simulink model "coefficent_aray"  (R2024a)
settings: Solver=FixedStepDiscrete  StartTime=0.0  StopTime=0.001  RelTol=1e-3
values from neighbouring files (symbols this model uses):
  Ts = 1/Fs    (= 7.50007500075e-06)    [new_generation_coeff.m]    (also in simon_test.m; simple_fft_test.m = 1/F; testPSD_c2d.m; testPSD_simulink.m)
settings Model: DataTypeOverride=Off  Creator=Simon  LastModifiedBy=Simon
settings OptimizationCC: BlockReduction=off  ConditionallyExecuteInputs=off  DefaultParameterBehavior=Inlined  InheritOutputTypeSmallerThanSingle=on
settings DebuggingCC: AlgebraicLoopMsg=error  SingleTaskRateTransMsg=error  UnconnectedInputMsg=warning  UnconnectedOutputMsg=warning  UnconnectedLineMsg=warning
settings HardwareCC: ProdBitPerPointer=32  ProdBitPerSizeT=32  ProdBitPerPtrDiffT=32  ProdLargestAtomicFloat=None  ProdIntDivRoundTo=Undefined  ProdEndianess=Unspecified  ProdWordSize=32  ProdHWDeviceType=ASIC/FPGA->ASIC/FPGA  TargetBitPerPointer=64  TargetBitPerSizeT=64  TargetBitPerPtrDiffT=64  TargetLongLongMode=on  TargetIntDivRoundTo=Zero  TargetEndianess=LittleEndian  TargetWordSize=64  TargetHWDeviceType=Custom Processor->MATLAB Host Computer  ProdEqTarget=off

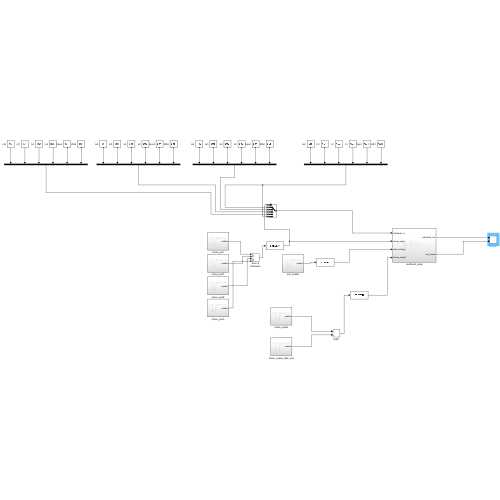
[thumbnail: Simulink's stored preview of the top-level diagram]
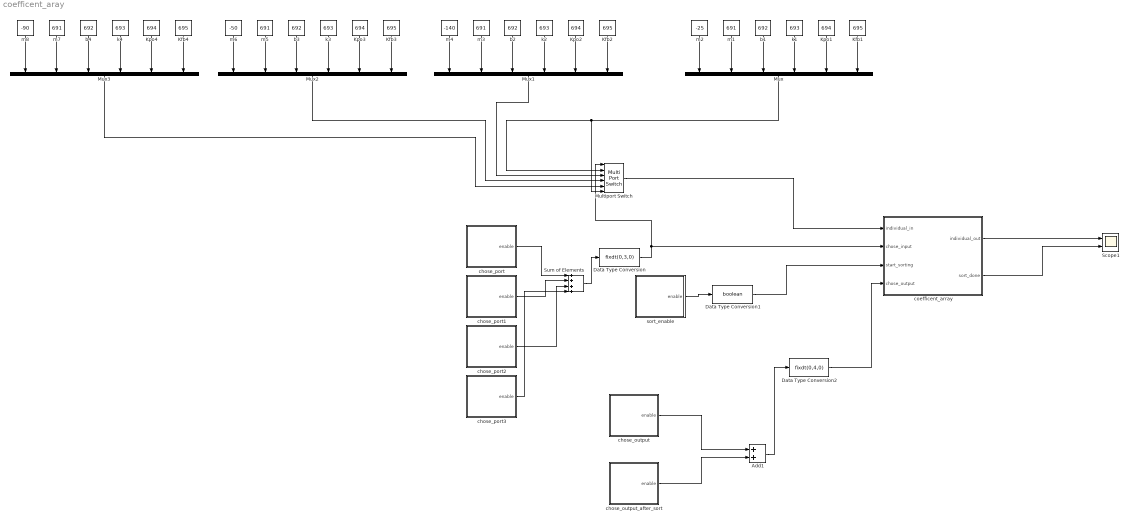
== system coefficent_aray ==
  Add1 : Sum
  Data Type Conversion : DataTypeConversion  OutDataTypeStr=fixdt(0,3,0)  SaturateOnIntegerOverflow=off  RndMeth=Floor
  Data Type Conversion1 : DataTypeConversion  OutDataTypeStr=boolean  SaturateOnIntegerOverflow=off  RndMeth=Floor
  Data Type Conversion2 : DataTypeConversion  OutDataTypeStr=fixdt(0,4,0)  SaturateOnIntegerOverflow=off  RndMeth=Floor
  Kfb{1..4} (4 alike) : Constant  Value=695  OutDataTypeStr=fixdt(1,64,32)  SampleTime=Ts
  Kpo{1..4} (4 alike) : Constant  Value=694  OutDataTypeStr=fixdt(1,64,32)  SampleTime=Ts
  Multiport Switch : MultiPortSwitch  Inputs=4  DataPortForDefault=Additional data port  DiagnosticForDefault=None  SaturateOnIntegerOverflow=off  InputSameDT=off
  Mux{,1..3} (4 alike) : Mux  Inputs=6
  Scope1 : Scope  NumInputPorts=2
  Sum of Elements : Sum  Inputs=++++
  b{1..4} (4 alike) : Constant  Value=692  OutDataTypeStr=fixdt(1,64,32)  SampleTime=Ts
  chose_output : Subsystem
  chose_output_after_sort : Subsystem
  chose_port : Subsystem
  chose_port1 : Subsystem
  chose_port2 : Subsystem
  chose_port3 : Subsystem
  coefficent_array : Subsystem
  k{1..4} (4 alike) : Constant  Value=693  OutDataTypeStr=fixdt(1,64,32)  SampleTime=Ts
  m{1,3,5,7} (4 alike) : Constant  Value=691  OutDataTypeStr=fixdt(1,64,32)  SampleTime=Ts
  m2 : Constant  Value=-25  OutDataTypeStr=fixdt(1,64,32)  SampleTime=Ts
  m4 : Constant  Value=-140  OutDataTypeStr=fixdt(1,64,32)  SampleTime=Ts
  m6 : Constant  Value=-50  OutDataTypeStr=fixdt(1,64,32)  SampleTime=Ts
  m8 : Constant  Value=-90  OutDataTypeStr=fixdt(1,64,32)  SampleTime=Ts
  sort_enable : Subsystem
  wires:
  Kpo1/1 -> Mux/5
  Kfb1/1 -> Mux/6
  k1/1 -> Mux/4
  m1/1 -> Mux/2
  b1/1 -> Mux/3
  m2/1 -> Mux/1
  chose_output/1(enable) -> Add1/1
  chose_output_after_sort/1(enable) -> Add1/2
  coefficent_array/1(individual_out) -> Scope1/1
  coefficent_array/2(sort_done) -> Scope1/2
  Kpo2/1 -> Mux1/5
  b2/1 -> Mux1/3
  k2/1 -> Mux1/4
  Kfb2/1 -> Mux1/6
  m4/1 -> Mux1/1
  m3/1 -> Mux1/2
  Kpo3/1 -> Mux2/5
  b3/1 -> Mux2/3
  k3/1 -> Mux2/4
  Kfb3/1 -> Mux2/6
  m6/1 -> Mux2/1
  m5/1 -> Mux2/2
  Kpo4/1 -> Mux3/5
  b4/1 -> Mux3/3
  k4/1 -> Mux3/4
  Kfb4/1 -> Mux3/6
  m8/1 -> Mux3/1
  m7/1 -> Mux3/2
  Multiport Switch/1 -> coefficent_array/1(individual_in)
  Mux/1 -> Multiport Switch/6, Multiport Switch/2
  Mux1/1 -> Multiport Switch/3
  Mux2/1 -> Multiport Switch/4
  Mux3/1 -> Multiport Switch/5
  chose_port/1(enable) -> Sum of Elements/1
  chose_port1/1(enable) -> Sum of Elements/2
  chose_port2/1(enable) -> Sum of Elements/3
  chose_port3/1(enable) -> Sum of Elements/4
  Add1/1 -> Data Type Conversion2/1
  sort_enable/1(enable) -> Data Type Conversion1/1
  Data Type Conversion/1 -> coefficent_array/2(chose_input), Multiport Switch/1
  Data Type Conversion1/1 -> coefficent_array/3(start_sorting)
  Data Type Conversion2/1 -> coefficent_array/4(chose_output)
  Sum of Elements/1 -> Data Type Conversion/1

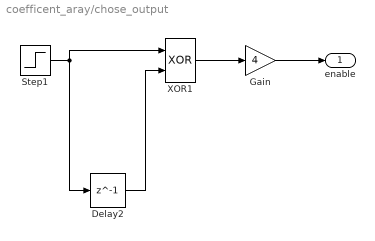
== system coefficent_aray/chose_output ==
  Delay2 : Delay  DelayLength=1  InitialCondition=0  SampleTime=Ts
  Gain : Gain  Gain=4
  Step1 : Step  Time=Ts*15  SampleTime=Ts
  XOR1 : Logic  Operator=XOR  IconShape=distinctive  AllPortsSameDT=off  OutDataTypeStr=fixdt(0,8)
  enable : Outport
  wires:
  XOR1/1 -> Gain/1
  Step1/1 -> Delay2/1, XOR1/1
  Delay2/1 -> XOR1/2
  Gain/1 -> enable/1

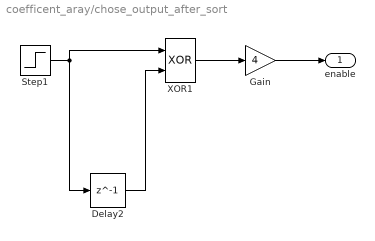
== system coefficent_aray/chose_output_after_sort ==
  Delay2 : Delay  DelayLength=1  InitialCondition=0  SampleTime=Ts
  Gain : Gain  Gain=4
  Step1 : Step  Time=Ts*50  SampleTime=Ts
  XOR1 : Logic  Operator=XOR  IconShape=distinctive  AllPortsSameDT=off  OutDataTypeStr=fixdt(0,8)
  enable : Outport
  wires:
  XOR1/1 -> Gain/1
  Step1/1 -> Delay2/1, XOR1/1
  Delay2/1 -> XOR1/2
  Gain/1 -> enable/1

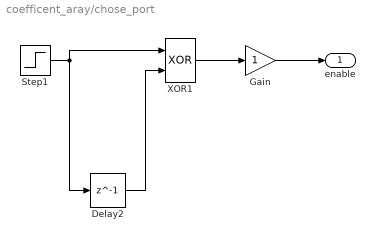
== system coefficent_aray/chose_port ==
  Delay2 : Delay  DelayLength=1  InitialCondition=0  SampleTime=Ts
  Gain : Gain
  Step1 : Step  Time=Ts*5  SampleTime=Ts
  XOR1 : Logic  Operator=XOR  IconShape=distinctive  AllPortsSameDT=off  OutDataTypeStr=fixdt(0,8)
  enable : Outport
  wires:
  XOR1/1 -> Gain/1
  Step1/1 -> Delay2/1, XOR1/1
  Delay2/1 -> XOR1/2
  Gain/1 -> enable/1

== system coefficent_aray/chose_port1 ==
  Delay2 : Delay  DelayLength=1  InitialCondition=0  SampleTime=Ts
  Gain : Gain  Gain=2
  Step1 : Step  Time=Ts*7  SampleTime=Ts
  XOR1 : Logic  Operator=XOR  IconShape=distinctive  AllPortsSameDT=off  OutDataTypeStr=fixdt(0,8)
  enable : Outport
  wires:
  XOR1/1 -> Gain/1
  Step1/1 -> Delay2/1, XOR1/1
  Delay2/1 -> XOR1/2
  Gain/1 -> enable/1

== system coefficent_aray/chose_port2 ==
  Delay2 : Delay  DelayLength=1  InitialCondition=0  SampleTime=Ts
  Gain : Gain  Gain=3
  Step1 : Step  Time=Ts*9  SampleTime=Ts
  XOR1 : Logic  Operator=XOR  IconShape=distinctive  AllPortsSameDT=off  OutDataTypeStr=fixdt(0,8)
  enable : Outport
  wires:
  XOR1/1 -> Gain/1
  Step1/1 -> Delay2/1, XOR1/1
  Delay2/1 -> XOR1/2
  Gain/1 -> enable/1

== system coefficent_aray/chose_port3 ==
  Delay2 : Delay  DelayLength=1  InitialCondition=0  SampleTime=Ts
  Gain : Gain  Gain=4
  Step1 : Step  Time=Ts*11  SampleTime=Ts
  XOR1 : Logic  Operator=XOR  IconShape=distinctive  AllPortsSameDT=off  OutDataTypeStr=fixdt(0,8)
  enable : Outport
  wires:
  XOR1/1 -> Gain/1
  Step1/1 -> Delay2/1, XOR1/1
  Delay2/1 -> XOR1/2
  Gain/1 -> enable/1

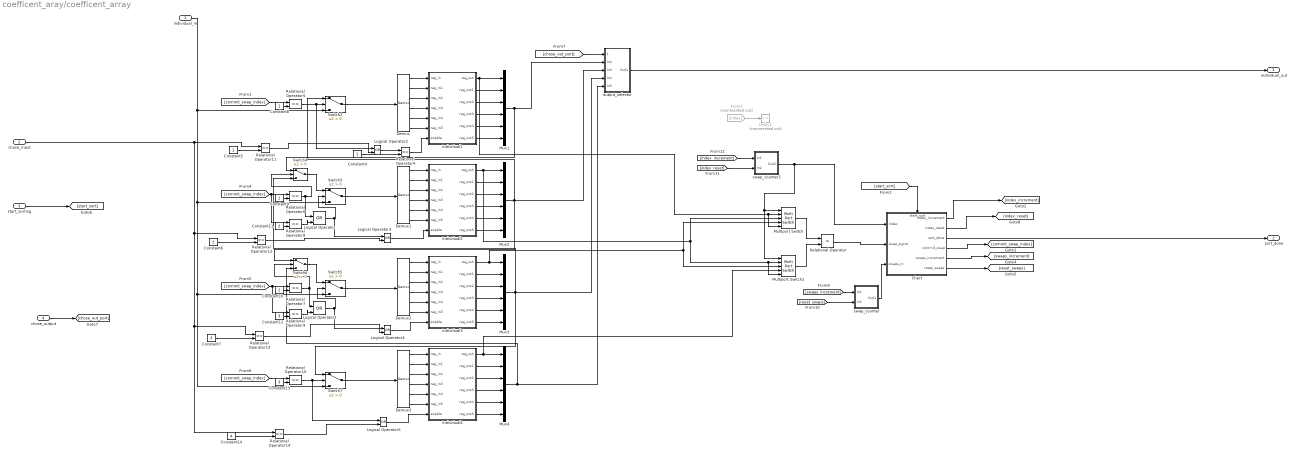
== system coefficent_aray/coefficent_array ==
  individual_in : Inport
  chose_input : Inport  Port=2
  start_sorting : Inport  Port=3
  chose_output : Inport  Port=4
  Chart : Stateflow chart  TreatAsAtomicUnit=on
      settings: PortSchema="{\"entries\":[{\"content\":{\"sides\":[{\"content\":{\"connectorIds\":[\"In1\",\"In4\",\"In3\"]},\"type\":\"ConnectorPlacement.EquallySpacedRectSide\",\"uuid\":\"bd2dafac-a5a9-4836-b8bd-cefb36fb6626\"},{\"content\":{\"connectorIds\":[\"Out1\",\"Out2\",\"Out3\",\"Out4\",\"Out5\",\"Out6\"],\"side\":\"RIGHT\"},\"type\":\"ConnectorPlacement.EquallySpacedRectSide\",\"uuid\":\"b2eb894e-8d56-4038-acbe-51c43d919a15\"},{\"content\":{\"connectorIds\":[\"In2\"],\"side\":\"TOP\"},\"type\":\"ConnectorPlacement.EquallySpacedRectSide\",\"uuid\":\"645ecb99-1eca-4a2d-8e44-d34ac75e3d1a\"}]},\"type\":\"ConnectorPlacement.EquallySpacedConnector\",\"uuid\":\"63f53eab-c5ec-482c-b992-d953653b0c27\"}],\"packageUris\":[\"http://schema.mathworks.com/mf0/Connector/R2020b\"],\"version\":\"1.0\"}"
  Constant10 : Constant  Value=2  OutDataTypeStr=fixdt(0,4,0)  SampleTime=Ts
  Constant11 : Constant  Value=2  OutDataTypeStr=fixdt(0,4,0)  SampleTime=Ts
  Constant12 : Constant  Value=3  OutDataTypeStr=fixdt(0,4,0)  SampleTime=Ts
  Constant13 : Constant  Value=3  OutDataTypeStr=fixdt(0,4,0)  SampleTime=Ts
  Constant14 : Constant  Value=4  OutDataTypeStr=fixdt(0,4,0)  SampleTime=Ts
  Constant{4..5,8..9} (4 alike) : Constant  OutDataTypeStr=fixdt(0,4,0)  SampleTime=Ts
  Constant6 : Constant  Value=2  OutDataTypeStr=fixdt(0,4,0)  SampleTime=Ts
  Constant7 : Constant  Value=3  OutDataTypeStr=fixdt(0,4,0)  SampleTime=Ts
  Delay1 : Delay  Commented=on  DelayLength=1  InitialCondition=0
  Demux{,1..3} (4 alike) : Demux  Outputs=6
  From3 : From  Commented=on  GotoTag=index
  Logical Operator{,1..5} (6 alike) : Logic  Operator=OR  IconShape=distinctive  AllPortsSameDT=off  OutDataTypeStr=boolean
  Multiport Switch : MultiPortSwitch  DataPortForDefault=Additional data port  DiagnosticForDefault=None  SaturateOnIntegerOverflow=off  InputSameDT=off
  Multiport Switch1 : MultiPortSwitch  DataPortForDefault=Additional data port  DiagnosticForDefault=None  SaturateOnIntegerOverflow=off  InputSameDT=off
  Mux{1..4} (4 alike) : Mux  Inputs=6
  Relational Operator : RelationalOperator  Operator=>  OutDataTypeStr=boolean  InputSameDT=off
  Relational Operator{4..14} (11 alike) : RelationalOperator  Operator===  OutDataTypeStr=boolean  RndMeth=Simplest  InputSameDT=off
  Switch{2..7} (6 alike) : Switch  Criteria=u2 > Threshold  SaturateOnIntegerOverflow=off  InputSameDT=off
  individual1 : Subsystem
  individual2 : Subsystem
  individual3 : Subsystem
  individual4 : Subsystem
  output_selector : Subsystem
  swap_counter : Subsystem
  swap_counter1 : Subsystem
  individual_out : Outport
  sort_done : Outport  Port=2
  wires:
  Logical Operator1/1 -> Logical Operator4/1, Switch5/2
  individual3/6(reg_out5) -> Mux3/6
  Constant9/1 -> Relational Operator6/2
  individual2/6(reg_out5) -> Mux2/6
  Demux2/3 -> individual3/3(reg_in2)
  Chart/5(swaps_increment) -> [swaps_increment]
  swap_counter1/1(Out1) -> Multiport Switch1/1, Multiport Switch/1, Chart/1(index)
  Switch4/1 -> Switch3/1
  individual1/1(reg_out) -> Mux1/1, Multiport Switch/5, Multiport Switch/2
  Demux/1 -> individual1/1(reg_in)
  Mux3/1 -> output_selector/4(In4), Switch7/1, Switch4/3
  individual3/3(reg_out2) -> Mux3/3
  individual4/4(reg_out3) -> Mux4/4
  Relational Operator10/1 -> Logical Operator5/1, Switch7/2
  [reset_swaps] -> swap_counter/2(In2)
  swap_counter/1(Out1) -> Chart/3(swaps_in)
  individual1/3(reg_out2) -> Mux1/3
  Relational Operator5/1 -> Logical Operator2/1, Switch2/2
  [swaps_increment] -> swap_counter/1(In1)
  [commit_swap_index] -> Relational Operator5/1
  Demux3/1 -> individual4/1(reg_in)
  Demux3/6 -> individual4/6(reg_in5)
  individual4/6(reg_out5) -> Mux4/6
  Demux1/4 -> individual2/4(reg_in3)
  Mux1/1 -> Switch4/1, output_selector/2(In2)
  Chart/6(reset_swaps) -> [reset_swaps]
  Relational Operator8/1 -> Logical Operator/2
  [commit_swap_index] -> Relational Operator8/1, Relational Operator6/1
  individual4/3(reg_out2) -> Mux4/3
  [commit_swap_index] -> Relational Operator9/1, Relational Operator7/1
  Logical Operator3/1 -> individual2/7(enable)
  Logical Operator5/1 -> individual4/7(enable)
  Multiport Switch/1 -> Relational Operator/1
  Constant11/1 -> Relational Operator8/2
  start_sorting/1 -> [start_sort]
  Chart/4(commit_swap) -> [commit_swap_index]
  Logical Operator/1 -> Logical Operator3/1, Switch3/2
  Demux/5 -> individual1/5(reg_in4)
  individual_in/1 -> Switch7/3, Switch5/3, Switch3/3, Switch2/3
  Demux2/1 -> individual3/1(reg_in)
  Switch3/1 -> Demux1/1
  individual4/1(reg_out) -> Multiport Switch1/4, Mux4/1
  Relational Operator6/1 -> Logical Operator/1, Switch4/2
  Constant4/1 -> Relational Operator4/2
  Constant13/1 -> Relational Operator10/2
  Constant12/1 -> Relational Operator9/2
  [commit_swap_index] -> Relational Operator10/1
  Demux2/4 -> individual3/4(reg_in3)
  individual2/4(reg_out3) -> Mux2/4
  Demux2/6 -> individual3/6(reg_in5)
  Demux1/6 -> individual2/6(reg_in5)
  Switch6/1 -> Switch5/1
  output_selector/1(Out1) -> individual_out/1
  Demux2/2 -> individual3/2(reg_in1)
  individual2/1(reg_out) -> Multiport Switch/3, Multiport Switch1/5, Multiport Switch1/2, Mux2/1
  Demux1/2 -> individual2/2(reg_in1)
  [chose_out_port] -> output_selector/1(chose_port)
  individual3/5(reg_out4) -> Mux3/5
  Demux/6 -> individual1/6(reg_in5)
  individual4/2(reg_out1) -> Mux4/2
  individual3/4(reg_out3) -> Mux3/4
  chose_input/1 -> Relational Operator14/1, Relational Operator13/1, Relational Operator12/1, Relational Operator11/1
  Relational Operator/1 -> Chart/4(swap_signal)
  Demux2/5 -> individual3/5(reg_in4)
  Logical Operator4/1 -> individual3/7(enable)
  Demux/3 -> individual1/3(reg_in2)
  Demux3/5 -> individual4/5(reg_in4)
  Demux3/4 -> individual4/4(reg_in3)
  Mux4/1 -> Switch6/3, output_selector/5(In5)
  Mux2/1 -> output_selector/3(In3), Switch6/1, Switch2/1
  individual3/1(reg_out) -> Multiport Switch1/3, Multiport Switch/4, Mux3/1
  individual4/5(reg_out4) -> Mux4/5
  individual3/2(reg_out1) -> Mux3/2
  individual2/5(reg_out4) -> Mux2/5
  Constant8/1 -> Relational Operator5/2
  Switch7/1 -> Demux3/1
  Chart/1(index_increment) -> [index_increment]
  Switch5/1 -> Demux2/1
  Demux3/2 -> individual4/2(reg_in1)
  individual2/2(reg_out1) -> Mux2/2
  Relational Operator7/1 -> Logical Operator1/1, Switch6/2
  Multiport Switch1/1 -> Relational Operator/2
  Demux1/5 -> individual2/5(reg_in4)
  Switch2/1 -> Demux/1
  Demux3/3 -> individual4/3(reg_in2)
  Relational Operator9/1 -> Logical Operator1/2
  Constant10/1 -> Relational Operator7/2
  Logical Operator2/1 -> Relational Operator4/1
  individual1/5(reg_out4) -> Mux1/5
  Demux/2 -> individual1/2(reg_in1)
  individual1/6(reg_out5) -> Mux1/6
  Relational Operator4/1 -> individual1/7(enable)
  individual1/2(reg_out1) -> Mux1/2
  Demux/4 -> individual1/4(reg_in3)
  Demux1/3 -> individual2/3(reg_in2)
  individual1/4(reg_out3) -> Mux1/4
  individual2/3(reg_out2) -> Mux2/3
  Demux1/1 -> individual2/1(reg_in)
  [start_sort] -> Chart/2(start_sort)
  Chart/3(sort_done) -> sort_done/1
  chose_output/1 -> [chose_out_port]
  Constant5/1 -> Relational Operator11/2
  Relational Operator11/1 -> Logical Operator2/2
  Constant6/1 -> Relational Operator12/2
  Relational Operator12/1 -> Logical Operator3/2
  Constant7/1 -> Relational Operator13/2
  Relational Operator13/1 -> Logical Operator4/2
  Relational Operator14/1 -> Logical Operator5/2
  Constant14/1 -> Relational Operator14/2
  [index_increment] -> swap_counter1/1(In1)
  [index_reset] -> swap_counter1/2(In2)
  From3/1 -> Delay1/1
  Chart/2(index_reset) -> [index_reset]

== system coefficent_aray/sort_enable ==
  Delay2 : Delay  DelayLength=1  InitialCondition=0  SampleTime=Ts
  Gain : Gain
  Step1 : Step  Time=Ts*20  SampleTime=Ts
  XOR1 : Logic  Operator=XOR  IconShape=distinctive  AllPortsSameDT=off  OutDataTypeStr=fixdt(0,8)
  enable : Outport
  wires:
  XOR1/1 -> Gain/1
  Step1/1 -> Delay2/1, XOR1/1
  Delay2/1 -> XOR1/2
  Gain/1 -> enable/1

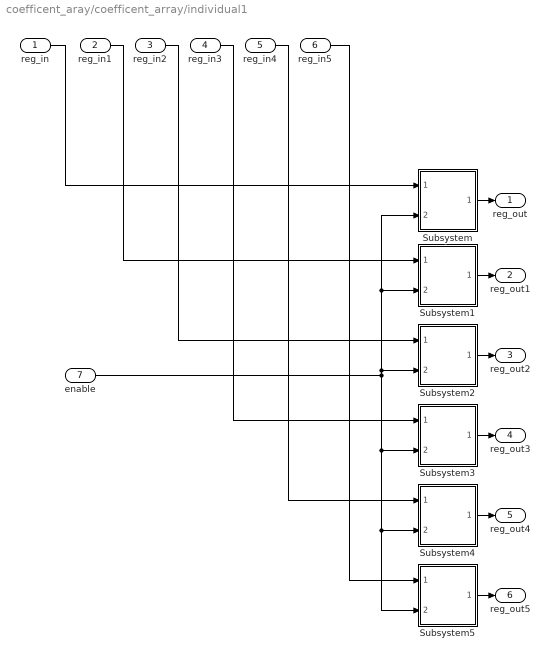
== system coefficent_aray/coefficent_array/individual1 ==
  reg_in : Inport
  reg_in1 : Inport  Port=2
  reg_in2 : Inport  Port=3
  reg_in3 : Inport  Port=4
  reg_in4 : Inport  Port=5
  reg_in5 : Inport  Port=6
  enable : Inport  Port=7
  Subsystem : Subsystem
  Subsystem1 : Subsystem
  Subsystem2 : Subsystem
  Subsystem3 : Subsystem
  Subsystem4 : Subsystem
  Subsystem5 : Subsystem
  reg_out : Outport
  reg_out1 : Outport  Port=2
  reg_out2 : Outport  Port=3
  reg_out3 : Outport  Port=4
  reg_out4 : Outport  Port=5
  reg_out5 : Outport  Port=6
  wires:
  enable/1 -> Subsystem2/2(enable), Subsystem1/2(enable), Subsystem/2(enable), Subsystem3/2(enable), Subsystem4/2(enable), Subsystem5/2(enable)
  Subsystem2/1(reg_out) -> reg_out2/1
  Subsystem4/1(reg_out) -> reg_out4/1
  Subsystem3/1(reg_out) -> reg_out3/1
  Subsystem1/1(reg_out) -> reg_out1/1
  reg_in/1 -> Subsystem/1(reg_in)
  Subsystem/1(reg_out) -> reg_out/1
  reg_in1/1 -> Subsystem1/1(reg_in)
  reg_in2/1 -> Subsystem2/1(reg_in)
  reg_in3/1 -> Subsystem3/1(reg_in)
  Subsystem5/1(reg_out) -> reg_out5/1
  reg_in4/1 -> Subsystem4/1(reg_in)
  reg_in5/1 -> Subsystem5/1(reg_in)

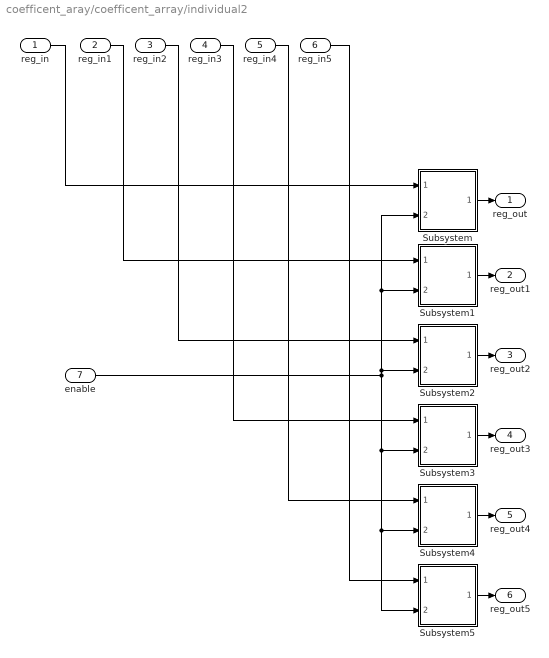
== system coefficent_aray/coefficent_array/individual2 ==
  reg_in : Inport
  reg_in1 : Inport  Port=2
  reg_in2 : Inport  Port=3
  reg_in3 : Inport  Port=4
  reg_in4 : Inport  Port=5
  reg_in5 : Inport  Port=6
  enable : Inport  Port=7
  Subsystem : Subsystem
  Subsystem1 : Subsystem
  Subsystem2 : Subsystem
  Subsystem3 : Subsystem
  Subsystem4 : Subsystem
  Subsystem5 : Subsystem
  reg_out : Outport
  reg_out1 : Outport  Port=2
  reg_out2 : Outport  Port=3
  reg_out3 : Outport  Port=4
  reg_out4 : Outport  Port=5
  reg_out5 : Outport  Port=6
  wires:
  enable/1 -> Subsystem2/2(enable), Subsystem1/2(enable), Subsystem/2(enable), Subsystem3/2(enable), Subsystem4/2(enable), Subsystem5/2(enable)
  Subsystem2/1(reg_out) -> reg_out2/1
  Subsystem4/1(reg_out) -> reg_out4/1
  Subsystem3/1(reg_out) -> reg_out3/1
  Subsystem1/1(reg_out) -> reg_out1/1
  reg_in/1 -> Subsystem/1(reg_in)
  Subsystem/1(reg_out) -> reg_out/1
  reg_in1/1 -> Subsystem1/1(reg_in)
  reg_in2/1 -> Subsystem2/1(reg_in)
  reg_in3/1 -> Subsystem3/1(reg_in)
  Subsystem5/1(reg_out) -> reg_out5/1
  reg_in4/1 -> Subsystem4/1(reg_in)
  reg_in5/1 -> Subsystem5/1(reg_in)

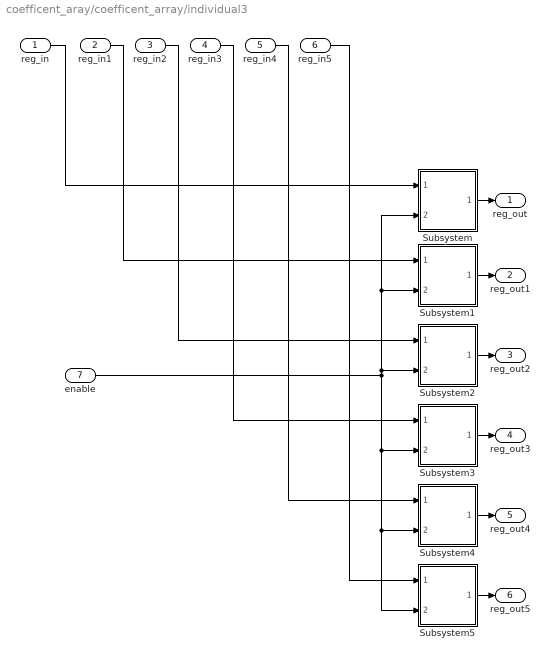
== system coefficent_aray/coefficent_array/individual3 ==
  reg_in : Inport
  reg_in1 : Inport  Port=2
  reg_in2 : Inport  Port=3
  reg_in3 : Inport  Port=4
  reg_in4 : Inport  Port=5
  reg_in5 : Inport  Port=6
  enable : Inport  Port=7
  Subsystem : Subsystem
  Subsystem1 : Subsystem
  Subsystem2 : Subsystem
  Subsystem3 : Subsystem
  Subsystem4 : Subsystem
  Subsystem5 : Subsystem
  reg_out : Outport
  reg_out1 : Outport  Port=2
  reg_out2 : Outport  Port=3
  reg_out3 : Outport  Port=4
  reg_out4 : Outport  Port=5
  reg_out5 : Outport  Port=6
  wires:
  enable/1 -> Subsystem2/2(enable), Subsystem1/2(enable), Subsystem/2(enable), Subsystem3/2(enable), Subsystem4/2(enable), Subsystem5/2(enable)
  Subsystem2/1(reg_out) -> reg_out2/1
  Subsystem4/1(reg_out) -> reg_out4/1
  Subsystem3/1(reg_out) -> reg_out3/1
  Subsystem1/1(reg_out) -> reg_out1/1
  reg_in/1 -> Subsystem/1(reg_in)
  Subsystem/1(reg_out) -> reg_out/1
  reg_in1/1 -> Subsystem1/1(reg_in)
  reg_in2/1 -> Subsystem2/1(reg_in)
  reg_in3/1 -> Subsystem3/1(reg_in)
  Subsystem5/1(reg_out) -> reg_out5/1
  reg_in4/1 -> Subsystem4/1(reg_in)
  reg_in5/1 -> Subsystem5/1(reg_in)

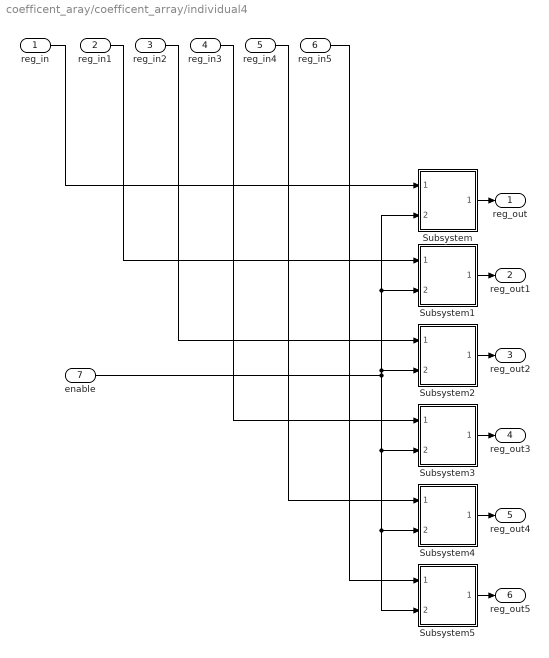
== system coefficent_aray/coefficent_array/individual4 ==
  reg_in : Inport
  reg_in1 : Inport  Port=2
  reg_in2 : Inport  Port=3
  reg_in3 : Inport  Port=4
  reg_in4 : Inport  Port=5
  reg_in5 : Inport  Port=6
  enable : Inport  Port=7
  Subsystem : Subsystem
  Subsystem1 : Subsystem
  Subsystem2 : Subsystem
  Subsystem3 : Subsystem
  Subsystem4 : Subsystem
  Subsystem5 : Subsystem
  reg_out : Outport
  reg_out1 : Outport  Port=2
  reg_out2 : Outport  Port=3
  reg_out3 : Outport  Port=4
  reg_out4 : Outport  Port=5
  reg_out5 : Outport  Port=6
  wires:
  enable/1 -> Subsystem2/2(enable), Subsystem1/2(enable), Subsystem/2(enable), Subsystem3/2(enable), Subsystem4/2(enable), Subsystem5/2(enable)
  Subsystem2/1(reg_out) -> reg_out2/1
  Subsystem4/1(reg_out) -> reg_out4/1
  Subsystem3/1(reg_out) -> reg_out3/1
  Subsystem1/1(reg_out) -> reg_out1/1
  reg_in/1 -> Subsystem/1(reg_in)
  Subsystem/1(reg_out) -> reg_out/1
  reg_in1/1 -> Subsystem1/1(reg_in)
  reg_in2/1 -> Subsystem2/1(reg_in)
  reg_in3/1 -> Subsystem3/1(reg_in)
  Subsystem5/1(reg_out) -> reg_out5/1
  reg_in4/1 -> Subsystem4/1(reg_in)
  reg_in5/1 -> Subsystem5/1(reg_in)

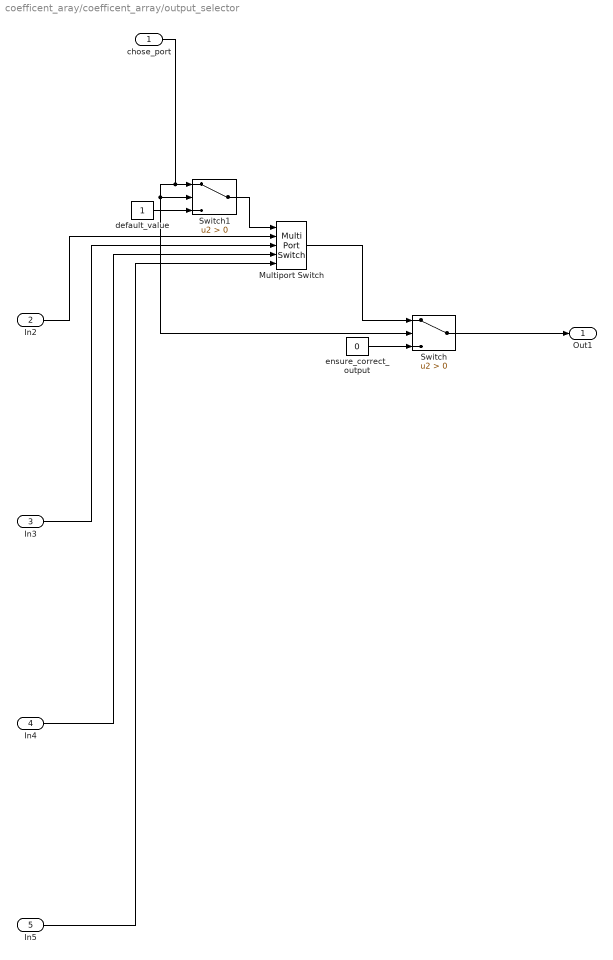
== system coefficent_aray/coefficent_array/output_selector ==
  chose_port : Inport
  In2 : Inport  Port=2
  In3 : Inport  Port=3
  In4 : Inport  Port=4
  In5 : Inport  Port=5
  Multiport Switch : MultiPortSwitch  Inputs=4  SaturateOnIntegerOverflow=off  InputSameDT=off
  Switch : Switch  Criteria=u2 > Threshold  SaturateOnIntegerOverflow=off  InputSameDT=off
  Switch1 : Switch  Criteria=u2 > Threshold  SaturateOnIntegerOverflow=off  InputSameDT=off
  default_value : Constant  OutDataTypeStr=fixdt(0,4,0)  SampleTime=Ts
  ensure_correct_output : Constant  Value=0  OutDataTypeStr=fixdt(0,1,0)  SampleTime=Ts
  Out1 : Outport
  wires:
  chose_port/1 -> Switch1/1, Switch/2, Switch1/2
  In2/1 -> Multiport Switch/2
  default_value/1 -> Switch1/3
  In4/1 -> Multiport Switch/4
  Multiport Switch/1 -> Switch/1
  Switch1/1 -> Multiport Switch/1
  In3/1 -> Multiport Switch/3
  ensure_correct_output/1 -> Switch/3
  Switch/1 -> Out1/1
  In5/1 -> Multiport Switch/5

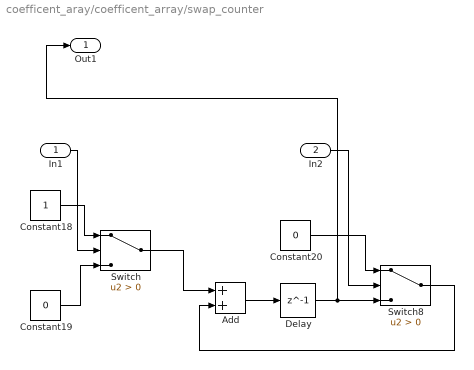
== system coefficent_aray/coefficent_array/swap_counter ==
  In1 : Inport
  In2 : Inport  Port=2
  Add : Sum  OutDataTypeStr=fixdt(0,4,0)  AccumDataTypeStr=fixdt(0,4,0)
  Constant18 : Constant  OutDataTypeStr=fixdt(0,4,0)  SampleTime=Ts
  Constant19 : Constant  Value=0  OutDataTypeStr=fixdt(0,4,0)  SampleTime=Ts
  Constant20 : Constant  Value=0  OutDataTypeStr=fixdt(0,4,0)  SampleTime=Ts
  Delay : Delay  DelayLength=1  InitialCondition=0  SampleTime=Ts
  Switch : Switch  Criteria=u2 > Threshold  OutDataTypeStr=fixdt(0,4,0)  SaturateOnIntegerOverflow=off  InputSameDT=off
  Switch8 : Switch  Criteria=u2 > Threshold  OutDataTypeStr=fixdt(0,4,0)  SaturateOnIntegerOverflow=off  InputSameDT=off
  Out1 : Outport
  wires:
  Constant19/1 -> Switch/3
  Switch8/1 -> Add/2
  Switch/1 -> Add/1
  Delay/1 -> Out1/1, Switch8/3
  In2/1 -> Switch8/2
  Add/1 -> Delay/1
  Constant20/1 -> Switch8/1
  Constant18/1 -> Switch/1
  In1/1 -> Switch/2

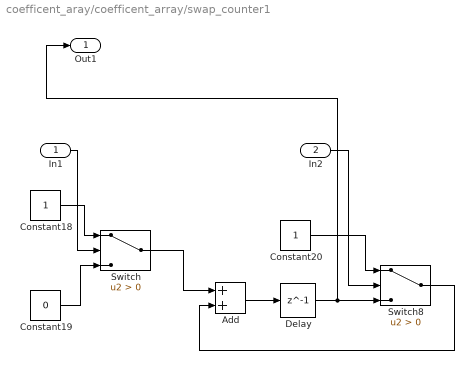
== system coefficent_aray/coefficent_array/swap_counter1 ==
  In1 : Inport
  In2 : Inport  Port=2
  Add : Sum  OutDataTypeStr=fixdt(0,4,0)  AccumDataTypeStr=fixdt(0,4,0)
  Constant18 : Constant  OutDataTypeStr=fixdt(0,4,0)  SampleTime=Ts
  Constant19 : Constant  Value=0  OutDataTypeStr=fixdt(0,4,0)  SampleTime=Ts
  Constant20 : Constant  OutDataTypeStr=fixdt(0,4,0)  SampleTime=Ts
  Delay : Delay  DelayLength=1  InitialCondition=0  SampleTime=Ts
  Switch : Switch  Criteria=u2 > Threshold  OutDataTypeStr=fixdt(0,4,0)  SaturateOnIntegerOverflow=off  InputSameDT=off
  Switch8 : Switch  Criteria=u2 > Threshold  OutDataTypeStr=fixdt(0,4,0)  SaturateOnIntegerOverflow=off  InputSameDT=off
  Out1 : Outport
  wires:
  Constant19/1 -> Switch/3
  Switch8/1 -> Add/2
  Switch/1 -> Add/1
  Delay/1 -> Out1/1, Switch8/3
  In2/1 -> Switch8/2
  Add/1 -> Delay/1
  Constant20/1 -> Switch8/1
  Constant18/1 -> Switch/1
  In1/1 -> Switch/2

== system coefficent_aray/coefficent_array/individual1/Subsystem ==
  reg_in : Inport
  enable : Inport  Port=2
  Delay : Delay  DelayLength=1  InitialCondition=0  SampleTime=Ts
  Switch : Switch  Criteria=u2 > Threshold  SaturateOnIntegerOverflow=off  InputSameDT=off
  reg_out : Outport
  wires:
  Delay/1 -> reg_out/1, Switch/3
  Switch/1 -> Delay/1
  enable/1 -> Switch/2
  reg_in/1 -> Switch/1

== system coefficent_aray/coefficent_array/individual1/Subsystem1 ==
  reg_in : Inport
  enable : Inport  Port=2
  Delay : Delay  DelayLength=1  InitialCondition=0  SampleTime=Ts
  Switch : Switch  Criteria=u2 > Threshold  SaturateOnIntegerOverflow=off  InputSameDT=off
  reg_out : Outport
  wires:
  Delay/1 -> reg_out/1, Switch/3
  Switch/1 -> Delay/1
  enable/1 -> Switch/2
  reg_in/1 -> Switch/1

== system coefficent_aray/coefficent_array/individual1/Subsystem2 ==
  reg_in : Inport
  enable : Inport  Port=2
  Delay : Delay  DelayLength=1  InitialCondition=0  SampleTime=Ts
  Switch : Switch  Criteria=u2 > Threshold  SaturateOnIntegerOverflow=off  InputSameDT=off
  reg_out : Outport
  wires:
  Delay/1 -> reg_out/1, Switch/3
  Switch/1 -> Delay/1
  enable/1 -> Switch/2
  reg_in/1 -> Switch/1

== system coefficent_aray/coefficent_array/individual1/Subsystem3 ==
  reg_in : Inport
  enable : Inport  Port=2
  Delay : Delay  DelayLength=1  InitialCondition=0  SampleTime=Ts
  Switch : Switch  Criteria=u2 > Threshold  SaturateOnIntegerOverflow=off  InputSameDT=off
  reg_out : Outport
  wires:
  Delay/1 -> reg_out/1, Switch/3
  Switch/1 -> Delay/1
  enable/1 -> Switch/2
  reg_in/1 -> Switch/1

== system coefficent_aray/coefficent_array/individual1/Subsystem4 ==
  reg_in : Inport
  enable : Inport  Port=2
  Delay : Delay  DelayLength=1  InitialCondition=0  SampleTime=Ts
  Switch : Switch  Criteria=u2 > Threshold  SaturateOnIntegerOverflow=off  InputSameDT=off
  reg_out : Outport
  wires:
  Delay/1 -> reg_out/1, Switch/3
  Switch/1 -> Delay/1
  enable/1 -> Switch/2
  reg_in/1 -> Switch/1

== system coefficent_aray/coefficent_array/individual1/Subsystem5 ==
  reg_in : Inport
  enable : Inport  Port=2
  Delay : Delay  DelayLength=1  InitialCondition=0  SampleTime=Ts
  Switch : Switch  Criteria=u2 > Threshold  SaturateOnIntegerOverflow=off  InputSameDT=off
  reg_out : Outport
  wires:
  Delay/1 -> reg_out/1, Switch/3
  Switch/1 -> Delay/1
  enable/1 -> Switch/2
  reg_in/1 -> Switch/1

== system coefficent_aray/coefficent_array/individual2/Subsystem ==
  reg_in : Inport
  enable : Inport  Port=2
  Delay : Delay  DelayLength=1  InitialCondition=0  SampleTime=Ts
  Switch : Switch  Criteria=u2 > Threshold  SaturateOnIntegerOverflow=off  InputSameDT=off
  reg_out : Outport
  wires:
  Delay/1 -> reg_out/1, Switch/3
  Switch/1 -> Delay/1
  enable/1 -> Switch/2
  reg_in/1 -> Switch/1

== system coefficent_aray/coefficent_array/individual2/Subsystem1 ==
  reg_in : Inport
  enable : Inport  Port=2
  Delay : Delay  DelayLength=1  InitialCondition=0  SampleTime=Ts
  Switch : Switch  Criteria=u2 > Threshold  SaturateOnIntegerOverflow=off  InputSameDT=off
  reg_out : Outport
  wires:
  Delay/1 -> reg_out/1, Switch/3
  Switch/1 -> Delay/1
  enable/1 -> Switch/2
  reg_in/1 -> Switch/1

== system coefficent_aray/coefficent_array/individual2/Subsystem2 ==
  reg_in : Inport
  enable : Inport  Port=2
  Delay : Delay  DelayLength=1  InitialCondition=0  SampleTime=Ts
  Switch : Switch  Criteria=u2 > Threshold  SaturateOnIntegerOverflow=off  InputSameDT=off
  reg_out : Outport
  wires:
  Delay/1 -> reg_out/1, Switch/3
  Switch/1 -> Delay/1
  enable/1 -> Switch/2
  reg_in/1 -> Switch/1

== system coefficent_aray/coefficent_array/individual2/Subsystem3 ==
  reg_in : Inport
  enable : Inport  Port=2
  Delay : Delay  DelayLength=1  InitialCondition=0  SampleTime=Ts
  Switch : Switch  Criteria=u2 > Threshold  SaturateOnIntegerOverflow=off  InputSameDT=off
  reg_out : Outport
  wires:
  Delay/1 -> reg_out/1, Switch/3
  Switch/1 -> Delay/1
  enable/1 -> Switch/2
  reg_in/1 -> Switch/1

== system coefficent_aray/coefficent_array/individual2/Subsystem4 ==
  reg_in : Inport
  enable : Inport  Port=2
  Delay : Delay  DelayLength=1  InitialCondition=0  SampleTime=Ts
  Switch : Switch  Criteria=u2 > Threshold  SaturateOnIntegerOverflow=off  InputSameDT=off
  reg_out : Outport
  wires:
  Delay/1 -> reg_out/1, Switch/3
  Switch/1 -> Delay/1
  enable/1 -> Switch/2
  reg_in/1 -> Switch/1

== system coefficent_aray/coefficent_array/individual2/Subsystem5 ==
  reg_in : Inport
  enable : Inport  Port=2
  Delay : Delay  DelayLength=1  InitialCondition=0  SampleTime=Ts
  Switch : Switch  Criteria=u2 > Threshold  SaturateOnIntegerOverflow=off  InputSameDT=off
  reg_out : Outport
  wires:
  Delay/1 -> reg_out/1, Switch/3
  Switch/1 -> Delay/1
  enable/1 -> Switch/2
  reg_in/1 -> Switch/1

== system coefficent_aray/coefficent_array/individual3/Subsystem ==
  reg_in : Inport
  enable : Inport  Port=2
  Delay : Delay  DelayLength=1  InitialCondition=0  SampleTime=Ts
  Switch : Switch  Criteria=u2 > Threshold  SaturateOnIntegerOverflow=off  InputSameDT=off
  reg_out : Outport
  wires:
  Delay/1 -> reg_out/1, Switch/3
  Switch/1 -> Delay/1
  enable/1 -> Switch/2
  reg_in/1 -> Switch/1

== system coefficent_aray/coefficent_array/individual3/Subsystem1 ==
  reg_in : Inport
  enable : Inport  Port=2
  Delay : Delay  DelayLength=1  InitialCondition=0  SampleTime=Ts
  Switch : Switch  Criteria=u2 > Threshold  SaturateOnIntegerOverflow=off  InputSameDT=off
  reg_out : Outport
  wires:
  Delay/1 -> reg_out/1, Switch/3
  Switch/1 -> Delay/1
  enable/1 -> Switch/2
  reg_in/1 -> Switch/1

== system coefficent_aray/coefficent_array/individual3/Subsystem2 ==
  reg_in : Inport
  enable : Inport  Port=2
  Delay : Delay  DelayLength=1  InitialCondition=0  SampleTime=Ts
  Switch : Switch  Criteria=u2 > Threshold  SaturateOnIntegerOverflow=off  InputSameDT=off
  reg_out : Outport
  wires:
  Delay/1 -> reg_out/1, Switch/3
  Switch/1 -> Delay/1
  enable/1 -> Switch/2
  reg_in/1 -> Switch/1

== system coefficent_aray/coefficent_array/individual3/Subsystem3 ==
  reg_in : Inport
  enable : Inport  Port=2
  Delay : Delay  DelayLength=1  InitialCondition=0  SampleTime=Ts
  Switch : Switch  Criteria=u2 > Threshold  SaturateOnIntegerOverflow=off  InputSameDT=off
  reg_out : Outport
  wires:
  Delay/1 -> reg_out/1, Switch/3
  Switch/1 -> Delay/1
  enable/1 -> Switch/2
  reg_in/1 -> Switch/1

== system coefficent_aray/coefficent_array/individual3/Subsystem4 ==
  reg_in : Inport
  enable : Inport  Port=2
  Delay : Delay  DelayLength=1  InitialCondition=0  SampleTime=Ts
  Switch : Switch  Criteria=u2 > Threshold  SaturateOnIntegerOverflow=off  InputSameDT=off
  reg_out : Outport
  wires:
  Delay/1 -> reg_out/1, Switch/3
  Switch/1 -> Delay/1
  enable/1 -> Switch/2
  reg_in/1 -> Switch/1

== system coefficent_aray/coefficent_array/individual3/Subsystem5 ==
  reg_in : Inport
  enable : Inport  Port=2
  Delay : Delay  DelayLength=1  InitialCondition=0  SampleTime=Ts
  Switch : Switch  Criteria=u2 > Threshold  SaturateOnIntegerOverflow=off  InputSameDT=off
  reg_out : Outport
  wires:
  Delay/1 -> reg_out/1, Switch/3
  Switch/1 -> Delay/1
  enable/1 -> Switch/2
  reg_in/1 -> Switch/1

== system coefficent_aray/coefficent_array/individual4/Subsystem ==
  reg_in : Inport
  enable : Inport  Port=2
  Delay : Delay  DelayLength=1  InitialCondition=0  SampleTime=Ts
  Switch : Switch  Criteria=u2 > Threshold  SaturateOnIntegerOverflow=off  InputSameDT=off
  reg_out : Outport
  wires:
  Delay/1 -> reg_out/1, Switch/3
  Switch/1 -> Delay/1
  enable/1 -> Switch/2
  reg_in/1 -> Switch/1

== system coefficent_aray/coefficent_array/individual4/Subsystem1 ==
  reg_in : Inport
  enable : Inport  Port=2
  Delay : Delay  DelayLength=1  InitialCondition=0  SampleTime=Ts
  Switch : Switch  Criteria=u2 > Threshold  SaturateOnIntegerOverflow=off  InputSameDT=off
  reg_out : Outport
  wires:
  Delay/1 -> reg_out/1, Switch/3
  Switch/1 -> Delay/1
  enable/1 -> Switch/2
  reg_in/1 -> Switch/1

== system coefficent_aray/coefficent_array/individual4/Subsystem2 ==
  reg_in : Inport
  enable : Inport  Port=2
  Delay : Delay  DelayLength=1  InitialCondition=0  SampleTime=Ts
  Switch : Switch  Criteria=u2 > Threshold  SaturateOnIntegerOverflow=off  InputSameDT=off
  reg_out : Outport
  wires:
  Delay/1 -> reg_out/1, Switch/3
  Switch/1 -> Delay/1
  enable/1 -> Switch/2
  reg_in/1 -> Switch/1

== system coefficent_aray/coefficent_array/individual4/Subsystem3 ==
  reg_in : Inport
  enable : Inport  Port=2
  Delay : Delay  DelayLength=1  InitialCondition=0  SampleTime=Ts
  Switch : Switch  Criteria=u2 > Threshold  SaturateOnIntegerOverflow=off  InputSameDT=off
  reg_out : Outport
  wires:
  Delay/1 -> reg_out/1, Switch/3
  Switch/1 -> Delay/1
  enable/1 -> Switch/2
  reg_in/1 -> Switch/1

== system coefficent_aray/coefficent_array/individual4/Subsystem4 ==
  reg_in : Inport
  enable : Inport  Port=2
  Delay : Delay  DelayLength=1  InitialCondition=0  SampleTime=Ts
  Switch : Switch  Criteria=u2 > Threshold  SaturateOnIntegerOverflow=off  InputSameDT=off
  reg_out : Outport
  wires:
  Delay/1 -> reg_out/1, Switch/3
  Switch/1 -> Delay/1
  enable/1 -> Switch/2
  reg_in/1 -> Switch/1

== system coefficent_aray/coefficent_array/individual4/Subsystem5 ==
  reg_in : Inport
  enable : Inport  Port=2
  Delay : Delay  DelayLength=1  InitialCondition=0  SampleTime=Ts
  Switch : Switch  Criteria=u2 > Threshold  SaturateOnIntegerOverflow=off  InputSameDT=off
  reg_out : Outport
  wires:
  Delay/1 -> reg_out/1, Switch/3
  Switch/1 -> Delay/1
  enable/1 -> Switch/2
  reg_in/1 -> Switch/1

== stateflow chart coefficent_aray/coefficent_array/Chart ==
  settings: executeAtInitialization=1
  state initial_sort
    during:
    index_increment = false;
    index_reset = true;
    swaps_increment = false;
    reset_swaps = true;
    sort_done = false;
  state round_increment
    entry:
    index_reset = true;
    reset_swaps = true;
  state not_perform_swap
    entry:
    commit_swap = 0;
  state start_round
    entry:
    reset_swaps = false;
    index_reset = false;
  state index_increment
    entry:
    index_increment = true;
    exit:
    index_increment = false;
  state perform_swap
    entry:
    commit_swap = index;
    swaps_increment = true;
    exit:
    commit_swap = 0;
    swaps_increment = false;
  state done_state
    entry:
    sort_done = true;
  (default) -> initial_sort
  done_state -> initial_sort
  initial_sort -> start_round : [start_sort]
  perform_swap -> round_increment [order 1] : [index == 3]
  not_perform_swap -> round_increment [order 3] : [index == 3]
  round_increment -> start_round
  start_round -> round_increment [order 2] : [index == 4]
  start_round -> not_perform_swap [order 1] : [swap_signal == false]
  not_perform_swap -> index_increment [order 1] : [index<3]
  not_perform_swap -> done_state [order 2] : [swaps_in == 0]
  start_round -> perform_swap [order 3] : [swap_signal == true]
  index_increment -> start_round
  perform_swap -> index_increment [order 2] : [index<3]
  data: index input; start_sort input; swaps_in input; index_increment output boolean; index_reset output boolean; sort_done output boolean; swap_signal input boolean; commit_swap output fixdt(0,4,0); swaps_increment output boolean; reset_swaps output boolean
